simulink model "MainDrive_Kuehlung_V1"  (Simulink 7.6)
settings: Solver=ode45  StartTime=0.0  StopTime=SimulTime  RelTol=1e-3
values from neighbouring files (symbols this model uses):
  R = 25    [ParamtersSpindel.m]    (also in PlottingSpindel.m = Scp_MainDriveT.signals(3).values(:,1)/1000; PlottingSpindel_Kuehlung.m = Scp_MainDriveT.signals(3).values(:,1)/1000)
  sb = 5.67*(10^-8)    (= 5.67e-08)    [ParamtersSpindel.m]
  T_amb = 295    [ParamtersSpindel.m]
undefined symbols (not defined in the file or in its folder): A, magnitude, MainDrive, MainDriveCooling
settings Model: Creator=Coni  LastModifiedBy=conid

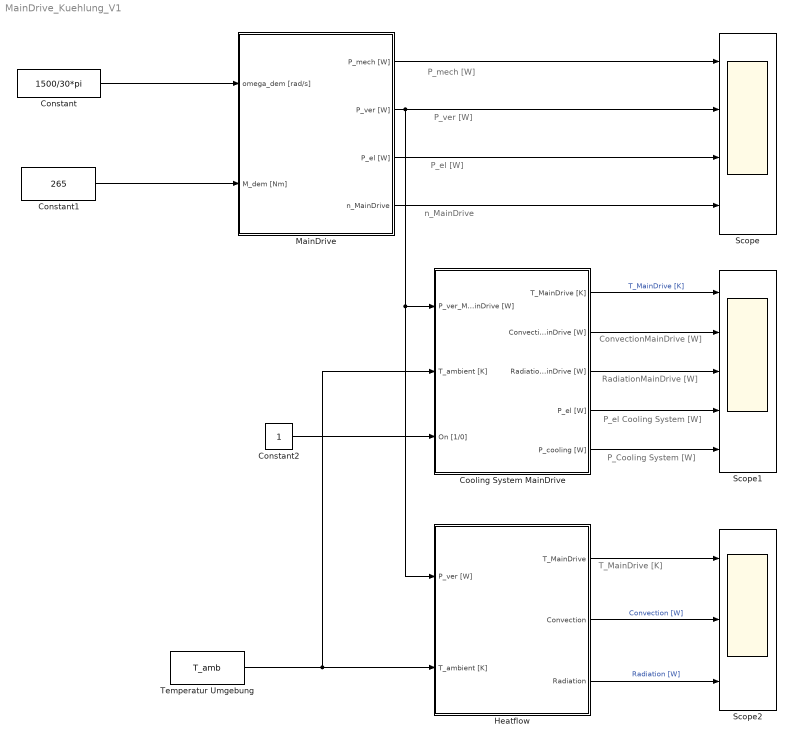
== system MainDrive_Kuehlung_V1 ==
  note: P_mech [W]
  note: P_ver [W]
  note: P_el [W]
  note: n_MainDrive
  note: T_MainDrive [K]
  note: ConvectionMainDrive [W]
  note: RadiationMainDrive [W]
  note: P_el Cooling System [W]
  note: P_Cooling System [W]
  Constant : Constant  Value=1500/30*pi
  Constant1 : Constant  Value=265
  Constant2 : Constant
  Cooling System MainDrive : Subsystem  TreatAsAtomicUnit=on
  Heatflow : Subsystem  TreatAsAtomicUnit=on
  MainDrive : Subsystem  TreatAsAtomicUnit=on
  Scope : Scope  NumInputPorts=4
      settings: TickLabels=on  TimeRange=100  YMin=0~-6e-010~-6e-010~-1.11022e-016  YMax=7e-026~-0~-0~-1.11022e-016  SaveName=Scp_MainDrive
  Scope1 : Scope  NumInputPorts=5
      settings: TickLabels=on  TimeRange=100  YMin=0~-5000~-2000~-0.1~-5  YMax=16000~30000~14000~0.9~5  SaveName=Scp_MainDrive1
  Scope2 : Scope  NumInputPorts=3
      settings: TickLabels=on  YMin=281.2~-1e-012~0  YMax=310.8~0~250  SaveName=Scp_MainDriveT
  Temperatur Umgebung : Constant  Value=T_amb
  wires:
  Constant/1 -> MainDrive/1(omega_dem [rad/s])
  Constant1/1 -> MainDrive/2(M_dem [Nm])
  MainDrive/1(P_mech [W]) -> Scope/1
  MainDrive/2(P_ver [W]) -> Scope/2, Heatflow/1(P_ver [W]), Cooling System MainDrive/1(P_ver_MainDrive [W])
  MainDrive/4(n_MainDrive) -> Scope/4
  Temperatur Umgebung/1 -> Heatflow/2(T_ambient [K]), Cooling System MainDrive/2(T_ambient [K])
  Heatflow/1(T_MainDrive) -> Scope2/1
  Heatflow/2(Convection) -> Scope2/2  "Convection [W]"
  Heatflow/3(Radiation) -> Scope2/3  "Radiation [W]"
  MainDrive/3(P_el [W]) -> Scope/3
  Cooling System MainDrive/1(T_MainDrive [K]) -> Scope1/1  "T_MainDrive [K]"
  Cooling System MainDrive/2(ConvectionMainDrive [W]) -> Scope1/2
  Cooling System MainDrive/3(RadiationMainDrive [W]) -> Scope1/3
  Cooling System MainDrive/4(P_el [W]) -> Scope1/4
  Cooling System MainDrive/5(P_cooling [W]) -> Scope1/5
  Constant2/1 -> Cooling System MainDrive/3(On [1/0])

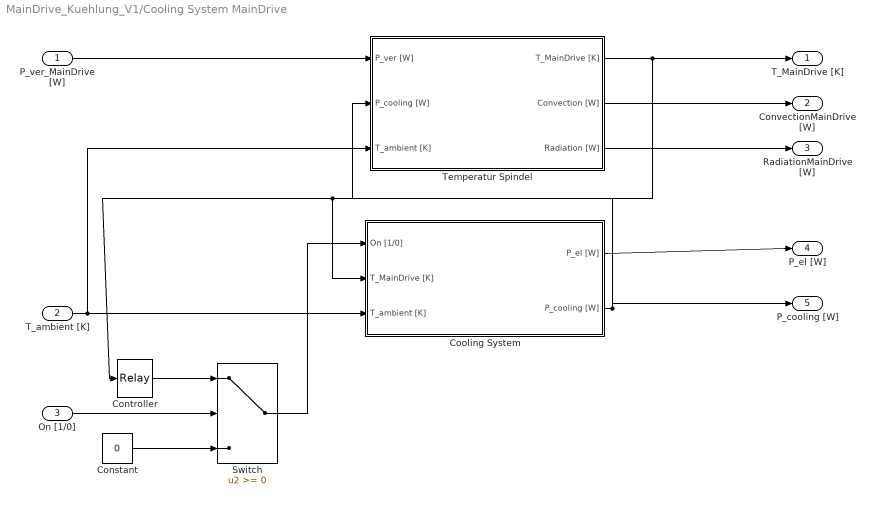
== system MainDrive_Kuehlung_V1/Cooling System MainDrive ==
  P_ver_MainDrive [W] : Inport
  T_ambient [K] : Inport  Port=2
  On [1/0] : Inport  Port=3
  Constant : Constant  Value=0
  Controller : Relay  OnSwitchValue=MainDriveCooling.Tmax  OffSwitchValue=MainDriveCooling.Tmin
  Cooling System : Subsystem
  Switch : Switch
  Temperatur Spindel : Subsystem
  T_MainDrive [K] : Outport
  ConvectionMainDrive [W] : Outport  Port=2
  RadiationMainDrive [W] : Outport  Port=3
  P_el [W] : Outport  Port=4
  P_cooling [W] : Outport  Port=5
  wires:
  P_ver_MainDrive [W]/1 -> Temperatur Spindel/1(P_ver [W])
  Constant/1 -> Switch/3
  On [1/0]/1 -> Switch/2
  Controller/1 -> Switch/1
  Temperatur Spindel/1(T_MainDrive [K]) -> Controller/1, Cooling System/2(T_MainDrive [K]), T_MainDrive [K]/1
  Switch/1 -> Cooling System/1(On [1/0])
  T_ambient [K]/1 -> Cooling System/3(T_ambient [K]), Temperatur Spindel/3(T_ambient [K])
  Cooling System/2(P_cooling [W]) -> Temperatur Spindel/2(P_cooling [W]), P_cooling [W]/1
  Temperatur Spindel/2(Convection [W]) -> ConvectionMainDrive [W]/1
  Temperatur Spindel/3(Radiation [W]) -> RadiationMainDrive [W]/1
  Cooling System/1(P_el [W]) -> P_el [W]/1

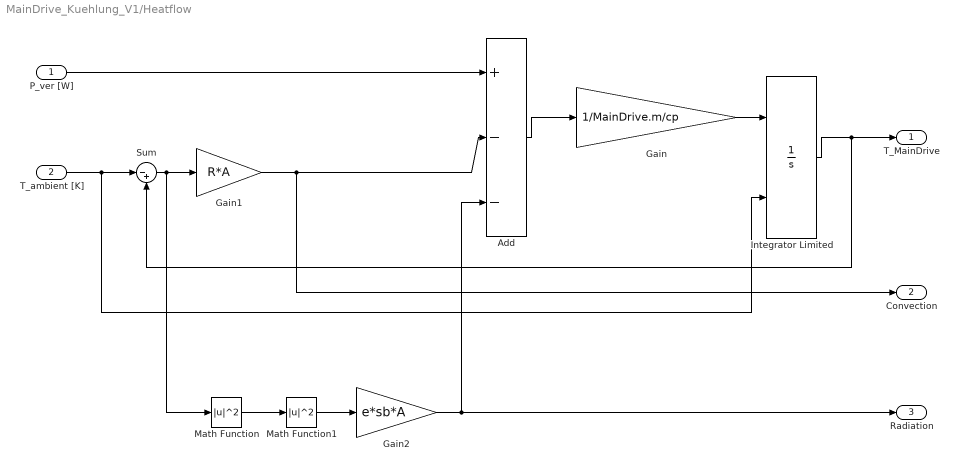
== system MainDrive_Kuehlung_V1/Heatflow ==
  P_ver [W] : Inport
  T_ambient [K] : Inport  Port=2
  Add : Sum  Inputs=+--
  Gain : Gain  Gain=1/MainDrive.m/cp
  Gain1 : Gain  Gain=R*A
  Gain2 : Gain  Gain=e*sb*A
  Integrator Limited : Integrator  InitialConditionSource=external  LimitOutput=on
  Math Function : Math  Operator=magnitude^2  SaturateOnIntegerOverflow=on
  Math Function1 : Math  Operator=magnitude^2  SaturateOnIntegerOverflow=on
  Sum : Sum  Inputs=|-+
  T_MainDrive : Outport
  Convection : Outport  Port=2
  Radiation : Outport  Port=3
  wires:
  P_ver [W]/1 -> Add/1
  T_ambient [K]/1 -> Sum/1, Integrator Limited/2
  Sum/1 -> Gain1/1, Math Function/1
  Gain/1 -> Integrator Limited/1
  Gain1/1 -> Add/2, Convection/1
  Integrator Limited/1 -> Sum/2, T_MainDrive/1
  Add/1 -> Gain/1
  Math Function/1 -> Math Function1/1
  Math Function1/1 -> Gain2/1
  Gain2/1 -> Add/3, Radiation/1

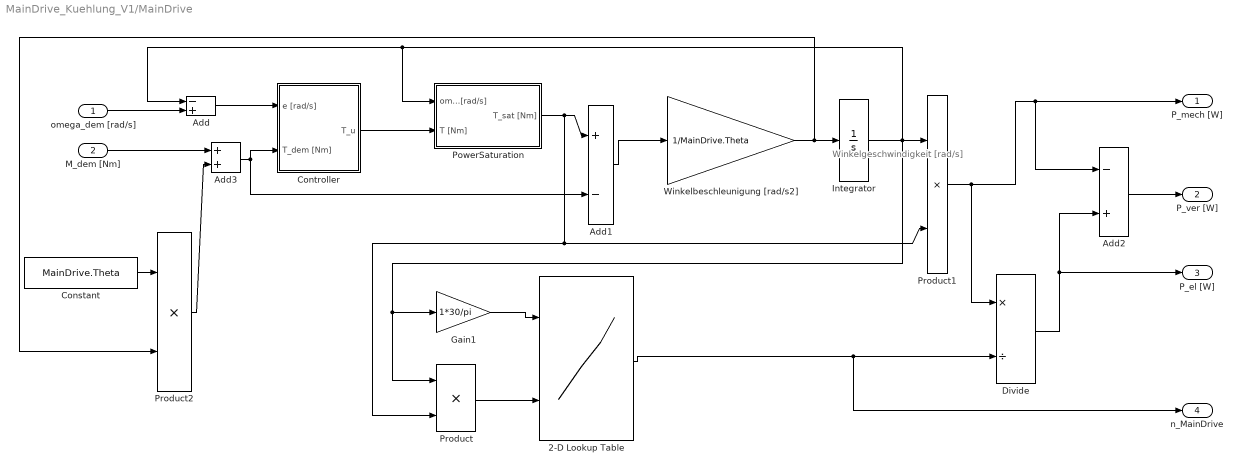
== system MainDrive_Kuehlung_V1/MainDrive ==
  note: Winkelgeschwindigkeit [rad/s]
  omega_dem [rad/s] : Inport
  M_dem [Nm] : Inport  Port=2
  2-D Lookup Table : Lookup_n-D  BreakpointsForDimension1=MainDrive.Tabelomega  BreakpointsForDimension2=MainDrive.TabelM  Table=MainDrive.Tabeleta  InterpMethod=Cubic spline  ExtrapMethod=Cubic spline  RndMeth=Simplest  InputSameDT=on
  Add : Sum  Inputs=-+
  Add1 : Sum  Inputs=+-
  Add2 : Sum  Inputs=-+
  Add3 : Sum
  Constant : Constant  Value=MainDrive.Theta
  Controller : Subsystem  TreatAsAtomicUnit=on
  Divide : Product  Inputs=*/
  Gain1 : Gain  Gain=1*30/pi
  Integrator : Integrator
  PowerSaturation : Subsystem  TreatAsAtomicUnit=on
  Product : Product  RndMeth=Zero
  Product1 : Product  RndMeth=Zero
  Product2 : Product  RndMeth=Zero
  Winkelbeschleunigung [rad/s2] : Gain  Gain=1/MainDrive.Theta
  P_mech [W] : Outport
  P_ver [W] : Outport  Port=2
  P_el [W] : Outport  Port=3
  n_MainDrive : Outport  Port=4
  wires:
  omega_dem [rad/s]/1 -> Add/2
  Add/1 -> Controller/1(e [rad/s])
  Controller/1(T_u) -> PowerSaturation/2(T [Nm])
  PowerSaturation/1(T_sat [Nm]) -> Add1/1, Product1/2, Product/2
  Add1/1 -> Winkelbeschleunigung [rad/s2]/1
  Winkelbeschleunigung [rad/s2]/1 -> Integrator/1, Product2/2
  Integrator/1 -> Product1/1, Add/1, PowerSaturation/1(omega [rad/s]), Product/1, Gain1/1
  Product1/1 -> Divide/1, P_mech [W]/1, Add2/1
  Add2/1 -> P_ver [W]/1
  Divide/1 -> Add2/2, P_el [W]/1
  2-D Lookup Table/1 -> Divide/2, n_MainDrive/1
  Product/1 -> 2-D Lookup Table/2
  Gain1/1 -> 2-D Lookup Table/1
  Constant/1 -> Product2/1
  Add3/1 -> Controller/2(T_dem [Nm]), Add1/2
  M_dem [Nm]/1 -> Add3/1
  Product2/1 -> Add3/2

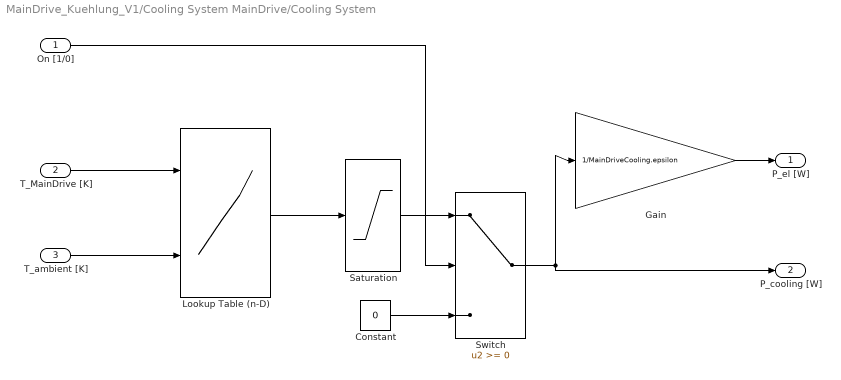
== system MainDrive_Kuehlung_V1/Cooling System MainDrive/Cooling System ==
  On [1/0] : Inport
  T_MainDrive [K] : Inport  Port=2
  T_ambient [K] : Inport  Port=3
  Constant : Constant  Value=0
  Gain : Gain  Gain=1/MainDriveCooling.epsilon
  Lookup Table (n-D) : Lookup_n-D  BreakpointsForDimension1=MainDriveCooling.Air.T_int  BreakpointsForDimension2=MainDriveCooling.Air.T_ext  Table=MainDriveCooling.Air.P  InterpMethod=Cubic spline  ExtrapMethod=None - Clip  InputSameDT=on
  Saturation : Saturate  UpperLimit=12000  LowerLimit=0
  Switch : Switch
  P_el [W] : Outport
  P_cooling [W] : Outport  Port=2
  wires:
  T_MainDrive [K]/1 -> Lookup Table (n-D)/1
  T_ambient [K]/1 -> Lookup Table (n-D)/2
  Constant/1 -> Switch/3
  On [1/0]/1 -> Switch/2
  Lookup Table (n-D)/1 -> Saturation/1
  Saturation/1 -> Switch/1
  Switch/1 -> Gain/1, P_cooling [W]/1
  Gain/1 -> P_el [W]/1

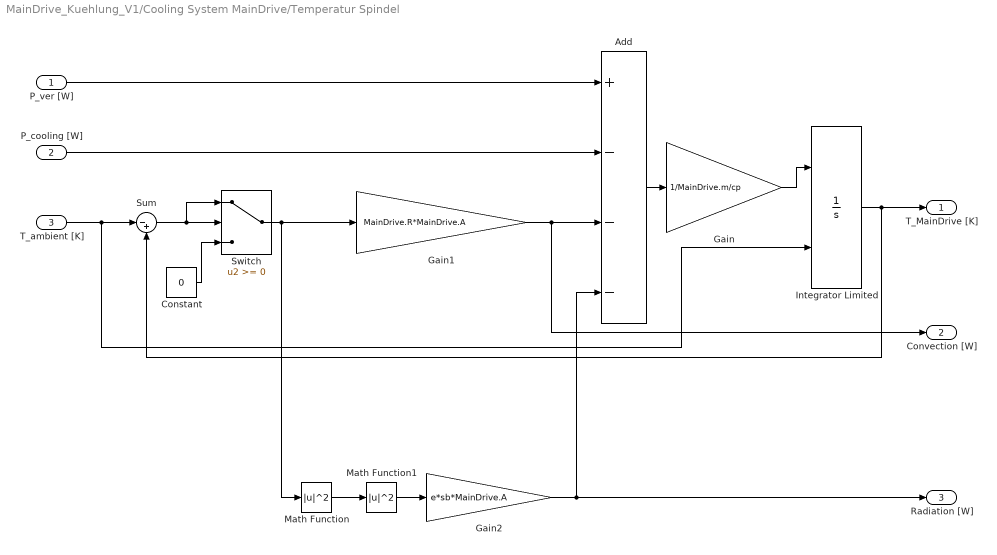
== system MainDrive_Kuehlung_V1/Cooling System MainDrive/Temperatur Spindel ==
  P_ver [W] : Inport
  P_cooling [W] : Inport  Port=2
  T_ambient [K] : Inport  Port=3
  Add : Sum  Inputs=+---
  Constant : Constant  Value=0
  Gain : Gain  Gain=1/MainDrive.m/cp
  Gain1 : Gain  Gain=MainDrive.R*MainDrive.A
  Gain2 : Gain  Gain=e*sb*MainDrive.A
  Integrator Limited : Integrator  InitialConditionSource=external  LimitOutput=on
  Math Function : Math  Operator=magnitude^2  SaturateOnIntegerOverflow=on
  Math Function1 : Math  Operator=magnitude^2  SaturateOnIntegerOverflow=on
  Sum : Sum  Inputs=|-+
  Switch : Switch
  T_MainDrive [K] : Outport
  Convection [W] : Outport  Port=2
  Radiation [W] : Outport  Port=3
  wires:
  P_ver [W]/1 -> Add/1
  Gain/1 -> Integrator Limited/1
  Gain1/1 -> Convection [W]/1, Add/3
  Integrator Limited/1 -> Sum/2, T_MainDrive [K]/1
  Add/1 -> Gain/1
  Math Function/1 -> Math Function1/1
  Math Function1/1 -> Gain2/1
  Gain2/1 -> Radiation [W]/1, Add/4
  P_cooling [W]/1 -> Add/2
  T_ambient [K]/1 -> Sum/1, Integrator Limited/2
  Switch/1 -> Gain1/1, Math Function/1
  Sum/1 -> Switch/2, Switch/1
  Constant/1 -> Switch/3

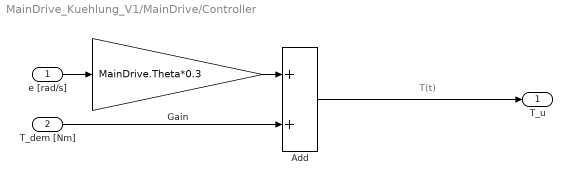
== system MainDrive_Kuehlung_V1/MainDrive/Controller ==
  note: T(t)
  e [rad/s] : Inport
  T_dem [Nm] : Inport  Port=2
  Add : Sum
  Gain : Gain  Gain=MainDrive.Theta*0.3
  T_u : Outport
  wires:
  Add/1 -> T_u/1
  T_dem [Nm]/1 -> Add/2
  Gain/1 -> Add/1
  e [rad/s]/1 -> Gain/1

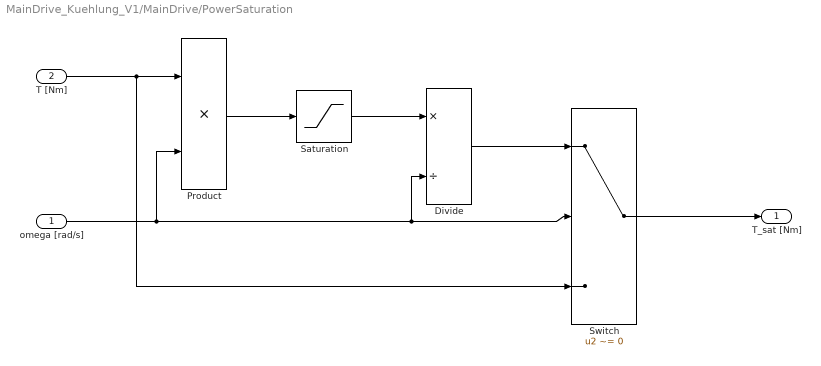
== system MainDrive_Kuehlung_V1/MainDrive/PowerSaturation ==
  omega [rad/s] : Inport
  T [Nm] : Inport  Port=2
  Divide : Product  Inputs=*/
  Product : Product  RndMeth=Zero
  Saturation : Saturate  UpperLimit=MainDrive.Pmax  LowerLimit=-MainDrive.Pmax
  Switch : Switch  Criteria=u2 ~= 0
  T_sat [Nm] : Outport
  wires:
  Product/1 -> Saturation/1
  Saturation/1 -> Divide/1
  Divide/1 -> Switch/1
  Switch/1 -> T_sat [Nm]/1
  T [Nm]/1 -> Product/1, Switch/3
  omega [rad/s]/1 -> Switch/2, Divide/2, Product/2
